simulink model "E1_Nonlinear"  (R2022a)
settings: Solver=VariableStepAuto  StartTime=0.0  StopTime=5  MaxStep=0.05  RelTol=1e-3
settings Model: Creator=Reza  LastModifiedBy=Reza

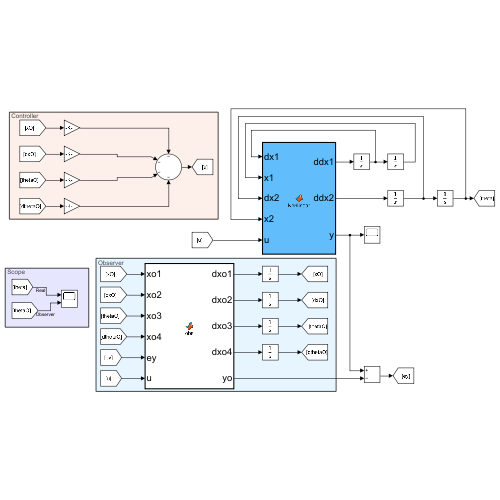
[thumbnail: Simulink's stored preview of the top-level diagram]
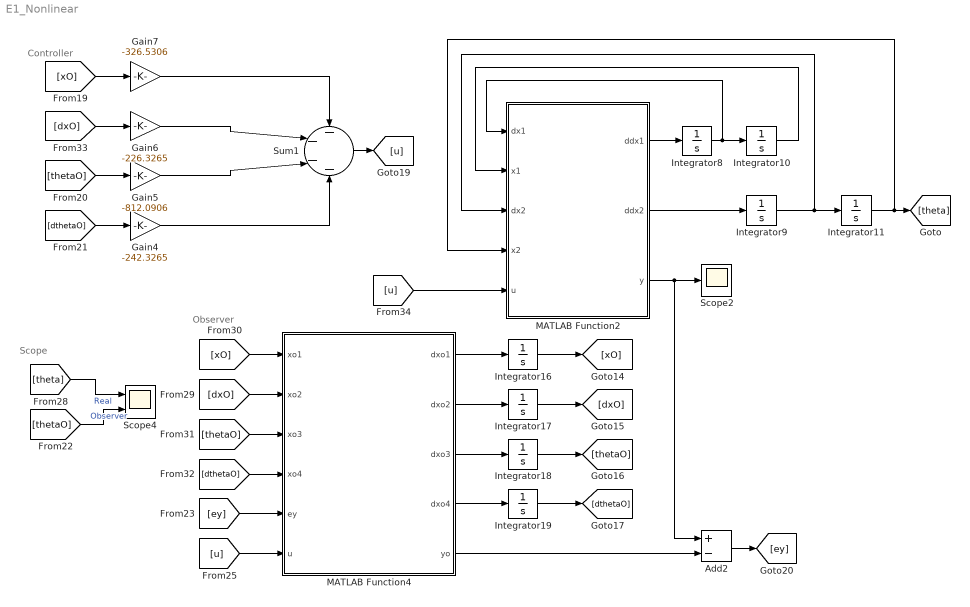
== system E1_Nonlinear ==
  note: Scope
  note: Controller
  note: Observer
  Add2 : Sum  Inputs=+-
  Gain4 : Gain  Gain=-242.3265
  Gain5 : Gain  Gain=-812.0906
  Gain6 : Gain  Gain=-226.3265
  Gain7 : Gain  Gain=-326.5306
  Integrator{8,10..11,16..19} (7 alike) : Integrator
  Integrator9 : Integrator  InitialCondition=10*pi/180
  MATLAB Function2 : MATLAB Function  TreatAsAtomicUnit=on
  MATLAB Function4 : MATLAB Function  TreatAsAtomicUnit=on
  Scope2 : Scope
  Scope4 : Scope  NumInputPorts=2
  Sum1 : Sum  Inputs=----
  wires:
  Add2/1 -> [ey]
  [u] -> MATLAB Function4/6(u)
  Integrator17/1 -> [dxO]
  Integrator18/1 -> [thetaO]
  Gain6/1 -> Sum1/2
  [ey] -> MATLAB Function4/5(ey)
  [thetaO] -> Scope4/2  "Observer"
  MATLAB Function2/3(y) -> Add2/1, Scope2/1
  MATLAB Function2/1(ddx1) -> Integrator8/1
  Integrator8/1 -> Integrator10/1, MATLAB Function2/1(dx1)
  Integrator10/1 -> MATLAB Function2/2(x1)
  Integrator11/1 -> [theta], MATLAB Function2/4(x2)
  [dthetaO] -> MATLAB Function4/4(xo4)
  [thetaO] -> Gain5/1
  [dxO] -> Gain6/1
  MATLAB Function2/2(ddx2) -> Integrator9/1
  Sum1/1 -> [u]
  MATLAB Function4/3(dxo3) -> Integrator18/1
  [xO] -> MATLAB Function4/1(xo1)
  [dthetaO] -> Gain4/1
  MATLAB Function4/5(yo) -> Add2/2
  Gain5/1 -> Sum1/3
  MATLAB Function4/4(dxo4) -> Integrator19/1
  Integrator16/1 -> [xO]
  MATLAB Function4/1(dxo1) -> Integrator16/1
  Integrator19/1 -> [dthetaO]
  [xO] -> Gain7/1
  [dxO] -> MATLAB Function4/2(xo2)
  [thetaO] -> MATLAB Function4/3(xo3)
  [theta] -> Scope4/1  "Real"
  MATLAB Function4/2(dxo2) -> Integrator17/1
  Gain4/1 -> Sum1/4
  [u] -> MATLAB Function2/5(u)
  Gain7/1 -> Sum1/1
  Integrator9/1 -> Integrator11/1, MATLAB Function2/3(dx2)

== matlab function E1_Nonlinear/MATLAB Function2 ==
  data: dx1 input; x1 input; dx2 input; x2 input; u input; ddx1 output; ddx2 output; y output
function [ddx1,ddx2,y] = Nonlinear(dx1,x1,dx2,x2,u)

M = 1;
m = 0.1;
l = 1;
g = 9.8;
k = 1;
R = 100;
r = 0.02;
M = [M+m m*l*cos(x2);cos(x2) l];
f = k/(R*r)*(u-k*dx1/r);
F = [f+m*l*dx2^2*sin(x2);g*sin(x2)];
ddx = inv(M)*F;
ddx1 = ddx(1);
ddx2 = ddx(2);
y = x1;

== matlab function E1_Nonlinear/MATLAB Function4 ==
  data: xo1 input; xo2 input; xo3 input; xo4 input; ey input; u input; dxo1 output; dxo2 output; dxo3 output; dxo4 output; yo output
function [dxo1,dxo2,dxo3,dxo4,yo] = obs(xo1,xo2,xo3,xo4,ey,u)


m = 0.1 ;
M = 1.0 ;
L = 1.0 ;
g = 10 ;
k = 1 ;
R = 100 ;
r = 0.02 ;

A = [ 0 ,           1           ,         0        , 0 ;
      0 ,   (-k^2/(M*R*r^2))    ,       -m*g/M     , 0 ;
      0 ,            0          ,         0        , 1 ;
      0 ,   (k^2/(M*R*r^2*L))   ,  ((M+m)*g/(M*L)) , 0 ] ;

B = [0 ; k/(M*R*r) ; 0 ;  -k/(M*R*r*L) ] ;

C = [ 1 , 0 , 0 , 0 ] ;

D = 0 ;

xo = [xo1;xo2;xo3;xo4];
L = [-11.9350;394.5103;-452.0058;-1993.6188];
dxo = A*xo+B*u+L*ey;
dxo1 = dxo(1);
dxo2 = dxo(2);
dxo3 = dxo(3);
dxo4 = dxo(4);
yo = C*xo+D*u;
